simulink model "BFE_TestHarness"  (Simulink 8.6)
settings: Solver=FixedStepDiscrete  StartTime=0.0  StopTime=3  FixedStep=Ts  RelTol=1e-3
PreLoadFcn:
  | addpath('MBD_Tests')
  | 
  | load('Workspace\EnvVar.mat')
  | run('MBD_Tests\MBD_tests_init.m')
  | if exist('tl_preloadfcn','file'), tl_preloadfcn(gcs,402); end
PostLoadFcn:
  | if exist('tl_postloadfcn','file'), tl_postloadfcn(gcs,402); end
InitFcn:
  | if exist('tlds_init','file'), tlds_init(gcs); end
StartFcn:
  | if exist('tlds_start','file'), tlds_start(gcs); end
StopFcn:
  | if exist('tlds_stop','file'), tlds_stop(gcs); end
undefined symbols (not defined in the file): ddv, Ts, u2, u3, u4
libraries: tllib x11, simulink x8, LIB_TF_G_111 x2, LIB_TF_G_12_StepControl x2, LIB_TF_G_112 x1, LIB_TF_G_113 x1
(part 2 of 17)

== system BFE_TestHarness/BFE_AC_BeltFunctionExecution/Subsystem/BFE_AC_BeltFunctionExecution/BFE_AC_BeltFunctionExecution/BFE_runExecuteEmergencyBrakingSequence ==
  u8MotorStageStatus_in : Inport  PortDimensions=1  mask(TL_Inport){data={'autosar',{'useautosarcommunication',1,'kind',3,'interrunnablevariable','u8MotorStageStatus'},'date',736809.44014567125}}
      settings: CopyFcn=if exist('tl_reset_reviewflag','file')==2,tl_reset_reviewflag(gcbh);end  DeleteFcn=if exist('delete_tlblock','file')==2,delete_tlblock(gcbh);end  NameChangeFcn=if exist('rename_tlblock','file')==2,rename_tlblock(gcbh);end  OpenFcn=if exist('tl_open_blockdlg','file')==2,tl_open_blockdlg(gcbh);else,open_system(gcbh,'parameter');end
      mask Help: eval(['if exist(''tl_online_help'',''file'') == 2, tl_online_help(''Topic'',''TL_Inport''),else, web([''jar:file:///'',matlabroot,''/help/toolbox/simulink/help.jar!/slref/' lower(get_param(gcbh,'Blocktype')) '.html''], ''-helpbrowser''),end'])
      mask Display: plot([0.2 0.35 NaN 0.65 0.8],[0 1 NaN 0 1]);
  s16MotorPowerOrder : Inport  Port=2  PortDimensions=1  mask(TL_Inport){data={'autosar',{'useautosarcommunication',1,'kind',3,'interrunnablevariable','s16MotorPowerOrder'},'date',736809.44014613423}}
      settings: CopyFcn=if exist('tl_reset_reviewflag','file')==2,tl_reset_reviewflag(gcbh);end  DeleteFcn=if exist('delete_tlblock','file')==2,delete_tlblock(gcbh);end  NameChangeFcn=if exist('rename_tlblock','file')==2,rename_tlblock(gcbh);end  OpenFcn=if exist('tl_open_blockdlg','file')==2,tl_open_blockdlg(gcbh);else,open_system(gcbh,'parameter');end
      mask Help: eval(['if exist(''tl_online_help'',''file'') == 2, tl_online_help(''Topic'',''TL_Inport''),else, web([''jar:file:///'',matlabroot,''/help/toolbox/simulink/help.jar!/slref/' lower(get_param(gcbh,'Blocktype')) '.html''], ''-helpbrowser''),end'])
      mask Display: plot([0.2 0.35 NaN 0.65 0.8],[0 1 NaN 0 1]);
  SSCP_pclMotorCurrent_ReadMotorCurrentInmA : Inport  Port=3  PortDimensions=1  mask(TL_Inport){data={'autosar',{'useautosarcommunication',1,'kind',4,'clientserverport','pclMotor_I','operation','Get_mA'},'date',735951.66862153937}}
      settings: CopyFcn=if exist('tl_reset_reviewflag','file')==2,tl_reset_reviewflag(gcbh);end  DeleteFcn=if exist('delete_tlblock','file')==2,delete_tlblock(gcbh);end  NameChangeFcn=if exist('rename_tlblock','file')==2,rename_tlblock(gcbh);end  OpenFcn=if exist('tl_open_blockdlg','file')==2,tl_open_blockdlg(gcbh);else,open_system(gcbh,'parameter');end
      mask Help: eval(['if exist(''tl_online_help'',''file'') == 2, tl_online_help(''Topic'',''TL_Inport''),else, web([''jar:file:///'',matlabroot,''/help/toolbox/simulink/help.jar!/slref/' lower(get_param(gcbh,'Blocktype')) '.html''], ''-helpbrowser''),end'])
      mask Display: plot([0.2 0.35 NaN 0.65 0.8],[0 1 NaN 0 1]);
  Trigger : TriggerPort  RequirementInfo={} %GIDa_b93913d7_0985_4350_88c4_327c5b9b98e8  TriggerType=function-call
  ANG regulation : Subsystem  TreatAsAtomicUnit=on
  Constant : Constant  Value=ddv('Common/KU8_ONE')  mask(TL_Constant){data={'output',{'variable','Common/KU8_ONE'},'date',735951.66860753472}}
      settings: CopyFcn=if exist('tl_reset_reviewflag','file')==2,tl_reset_reviewflag(gcbh);end  DeleteFcn=if exist('delete_tlblock','file')==2,delete_tlblock(gcbh);end  NameChangeFcn=if exist('rename_tlblock','file')==2,rename_tlblock(gcbh);end  OpenFcn=if exist('tl_open_blockdlg','file')==2,tl_open_blockdlg(gcbh);else,open_system(gcbh,'parameter');end
      mask Help: eval(['if exist(''tl_online_help'',''file'') == 2, tl_online_help(''Topic'',''TL_Constant''),else, web([''jar:file:///'',matlabroot,''/help/toolbox/simulink/help.jar!/slref/' lower(get_param(gcbh,'Blocktype')) '.html''], ''-helpbrowser''),end'])
      mask Display: plot([-0.05, 1.05, NaN, -0.05, 1.05],[.01, .01, NaN, .99, .99])
  Constant1 : Constant  Value=ddv('EmergencyBraking/CAL_KU16_PYRO_SEQ_BRAKING_DURATION')  SampleTime=-1  mask(TL_Constant){data={'output',{'variable','EmergencyBraking/CAL_KU16_PYRO_SEQ_BRAKING_DURATION'},'date',735951.66860717593}}
      settings: CopyFcn=if exist('tl_reset_reviewflag','file')==2,tl_reset_reviewflag(gcbh);end  DeleteFcn=if exist('delete_tlblock','file')==2,delete_tlblock(gcbh);end  NameChangeFcn=if exist('rename_tlblock','file')==2,rename_tlblock(gcbh);end  OpenFcn=if exist('tl_open_blockdlg','file')==2,tl_open_blockdlg(gcbh);else,open_system(gcbh,'parameter');end
      mask Help: eval(['if exist(''tl_online_help'',''file'') == 2, tl_online_help(''Topic'',''TL_Constant''),else, web([''jar:file:///'',matlabroot,''/help/toolbox/simulink/help.jar!/slref/' lower(get_param(gcbh,'Blocktype')) '.html''], ''-helpbrowser''),end'])
      mask Display: plot([-0.05, 1.05, NaN, -0.05, 1.05],[.01, .01, NaN, .99, .99])
  Constant2 : Constant  Value=ddv('Common/KU16_ZERO')  mask(TL_Constant){data={'output',{'variable','Common/KU16_ZERO'},'date',735951.6686068055}}
      settings: CopyFcn=if exist('tl_reset_reviewflag','file')==2,tl_reset_reviewflag(gcbh);end  DeleteFcn=if exist('delete_tlblock','file')==2,delete_tlblock(gcbh);end  NameChangeFcn=if exist('rename_tlblock','file')==2,rename_tlblock(gcbh);end  OpenFcn=if exist('tl_open_blockdlg','file')==2,tl_open_blockdlg(gcbh);else,open_system(gcbh,'parameter');end
      mask Help: eval(['if exist(''tl_online_help'',''file'') == 2, tl_online_help(''Topic'',''TL_Constant''),else, web([''jar:file:///'',matlabroot,''/help/toolbox/simulink/help.jar!/slref/' lower(get_param(gcbh,'Blocktype')) '.html''], ''-helpbrowser''),end'])
      mask Display: plot([-0.05, 1.05, NaN, -0.05, 1.05],[.01, .01, NaN, .99, .99])
  Idle State : Subsystem  TreatAsAtomicUnit=on
  If : If  IfExpression=u1
  Relational Operator : RelationalOperator  Operator=~=  OutDataTypeStr=boolean  mask(TL_RelationalOperator){data={'date',735951.66860112268}}
      settings: DeleteFcn=if exist('delete_tlblock','file')==2,delete_tlblock(gcbh);end  NameChangeFcn=if exist('rename_tlblock','file')==2,rename_tlblock(gcbh);end  OpenFcn=if exist('tl_open_blockdlg','file')==2,tl_open_blockdlg(gcbh);else,open_system(gcbh,'parameter');end
      mask Help: eval(['if exist(''tl_online_help'',''file'') == 2, tl_online_help(''Topic'',''TL_RelationalOperator''),else, web([''jar:file:///'',matlabroot,''/help/toolbox/simulink/help.jar!/slref/' lower(get_param(gcbh,'Blocktype')) '.html''], ''-helpbrowser''),end'])
      mask Display: plot([-0.05, 1.05, NaN, -0.05, 1.05],[.01, .01, NaN, .99, .99])
  Relational Operator1 : RelationalOperator  Operator=>  OutDataTypeStr=boolean  mask(TL_RelationalOperator){data={'output',{'name','bIsFirstPhaseFinished'},'date',735951.66860086808}}
      settings: DeleteFcn=if exist('delete_tlblock','file')==2,delete_tlblock(gcbh);end  NameChangeFcn=if exist('rename_tlblock','file')==2,rename_tlblock(gcbh);end  OpenFcn=if exist('tl_open_blockdlg','file')==2,tl_open_blockdlg(gcbh);else,open_system(gcbh,'parameter');end
      mask Help: eval(['if exist(''tl_online_help'',''file'') == 2, tl_online_help(''Topic'',''TL_RelationalOperator''),else, web([''jar:file:///'',matlabroot,''/help/toolbox/simulink/help.jar!/slref/' lower(get_param(gcbh,'Blocktype')) '.html''], ''-helpbrowser''),end'])
      mask Display: plot([-0.05, 1.05, NaN, -0.05, 1.05],[.01, .01, NaN, .99, .99])
  Runnable : tllib/Function  data={'autosar',{'useautosarspecification',1,'softwarecomponent','AUTOLIV/SoftwareComponents/BFE/BFE_AC_BeltFunctionExecution','runnable','BFE_runExecuteEmergencyBrakingSequence'},'date',736809.44014254631}  displayString=RUNNABLE
  Sum : Sum  mask(TL_Sum){data={'output',{'name','u16LocalCounter','type','UInt16','checkmin',1,'checkmax',1},'date',735951.66860057868}}
      settings: CopyFcn=if exist('tl_reset_reviewflag','file')==2,tl_reset_reviewflag(gcbh);end  DeleteFcn=if exist('delete_tlblock','file')==2,delete_tlblock(gcbh);end  NameChangeFcn=if exist('rename_tlblock','file')==2,rename_tlblock(gcbh);end  OpenFcn=if exist('tl_open_blockdlg','file')==2,tl_open_blockdlg(gcbh);else,open_system(gcbh,'parameter');end
      mask Help: eval(['if exist(''tl_online_help'',''file'') == 2, tl_online_help(''Topic'',''TL_Sum''),else, web([''jar:file:///'',matlabroot,''/help/toolbox/simulink/help.jar!/slref/' lower(get_param(gcbh,'Blocktype')) '.html''], ''-helpbrowser''),end'])
      mask Display: plot([-0.05, 1.05, NaN, -0.05, 1.05],[.01, .01, NaN, .99, .99])
  Switch : Switch  Criteria=u2 ~= 0  mask(TL_Switch){data={'output',{'name','u16FilteredPrevCounterECPL','type','UInt16'},'date',735951.66860002314}}
      settings: CopyFcn=if exist('tl_reset_reviewflag','file')==2,tl_reset_reviewflag(gcbh);end  DeleteFcn=if exist('delete_tlblock','file')==2,delete_tlblock(gcbh);end  NameChangeFcn=if exist('rename_tlblock','file')==2,rename_tlblock(gcbh);end  OpenFcn=if exist('tl_open_blockdlg','file')==2,tl_open_blockdlg(gcbh);else,open_system(gcbh,'parameter');end
      mask Help: eval(['if exist(''tl_online_help'',''file'') == 2, tl_online_help(''Topic'',''TL_Switch''),else, web([''jar:file:///'',matlabroot,''/help/toolbox/simulink/help.jar!/slref/' lower(get_param(gcbh,'Blocktype')) '.html''], ''-helpbrowser''),end'])
      mask Display: plot([-0.05, 1.05, NaN, -0.05, 1.05],[.01, .01, NaN, .99, .99])
  Unit Delay : UnitDelay  SampleTime=-1  mask(TL_UnitDelay){data={'output',{'type','UInt16'},'state',{'name','u16CounterEmergencySeq','type','UInt16'},'date',735951.6685995023}}
      settings: CopyFcn=if exist('tl_reset_reviewflag','file')==2,tl_reset_reviewflag(gcbh);end  DeleteFcn=if exist('delete_tlblock','file')==2,delete_tlblock(gcbh);end  NameChangeFcn=if exist('rename_tlblock','file')==2,rename_tlblock(gcbh);end  OpenFcn=if exist('tl_open_blockdlg','file')==2,tl_open_blockdlg(gcbh);else,open_system(gcbh,'parameter');end
      mask Help: eval(['if exist(''tl_online_help'',''file'') == 2, tl_online_help(''Topic'',''TL_UnitDelay''),else, web([''jar:file:///'',matlabroot,''/help/toolbox/simulink/help.jar!/slref/' lower(get_param(gcbh,'Blocktype')) '.html''], ''-helpbrowser''),end'])
      mask Display: plot([-0.05, 1.05, NaN, -0.05, 1.05],[.01, .01, NaN, .99, .99])
  Unit Delay1 : UnitDelay  InitialCondition=170  SampleTime=-1  mask(TL_UnitDelay){data={'output',{'type','UInt8'},'state',{'name','u8PrevMotorStageStatus','type','UInt8'},'date',735951.66859895829}}
      settings: CopyFcn=if exist('tl_reset_reviewflag','file')==2,tl_reset_reviewflag(gcbh);end  DeleteFcn=if exist('delete_tlblock','file')==2,delete_tlblock(gcbh);end  NameChangeFcn=if exist('rename_tlblock','file')==2,rename_tlblock(gcbh);end  OpenFcn=if exist('tl_open_blockdlg','file')==2,tl_open_blockdlg(gcbh);else,open_system(gcbh,'parameter');end
      mask Help: eval(['if exist(''tl_online_help'',''file'') == 2, tl_online_help(''Topic'',''TL_UnitDelay''),else, web([''jar:file:///'',matlabroot,''/help/toolbox/simulink/help.jar!/slref/' lower(get_param(gcbh,'Blocktype')) '.html''], ''-helpbrowser''),end'])
      mask Display: plot([-0.05, 1.05, NaN, -0.05, 1.05],[.01, .01, NaN, .99, .99])
  terminator{2..5} (4 alike) : Terminator
  u8MotorStageStatus : Merge  mask(TL_Merge){data={'output',{'name','$B'},'date',735951.66859842592}}
      settings: CopyFcn=if exist('tl_reset_reviewflag','file')==2,tl_reset_reviewflag(gcbh);end  DeleteFcn=if exist('delete_tlblock','file')==2,delete_tlblock(gcbh);end  NameChangeFcn=if exist('rename_tlblock','file')==2,rename_tlblock(gcbh);end  OpenFcn=if exist('tl_open_blockdlg','file')==2,tl_open_blockdlg(gcbh);else,open_system(gcbh,'parameter');end
      mask Help: eval(['if exist(''tl_online_help'',''file'') == 2, tl_online_help(''Topic'',''TL_Merge''),else, web([''jar:file:///'',matlabroot,''/help/toolbox/simulink/help.jar!/slref/' lower(get_param(gcbh,'Blocktype')) '.html''], ''-helpbrowser''),end'])
      mask Display: plot([-0.05, 1.05, NaN, -0.05, 1.05],[.01, .01, NaN, .99, .99])
  u8MotorStageStatus_out : Outport  PortDimensions=1  InitialOutput=170  mask(TL_Outport){data={'autosar',{'useautosarcommunication',1,'kind',3,'communicationmode',1,'interrunnablevariable','u8MotorStageStatus'},'date',736809.4401464815}}
      settings: CopyFcn=if exist('tl_reset_reviewflag','file')==2,tl_reset_reviewflag(gcbh);end  DeleteFcn=if exist('delete_tlblock','file')==2,delete_tlblock(gcbh);end  NameChangeFcn=if exist('rename_tlblock','file')==2,rename_tlblock(gcbh);end  OpenFcn=if exist('tl_open_blockdlg','file')==2,tl_open_blockdlg(gcbh);else,open_system(gcbh,'parameter');end
      mask Help: eval(['if exist(''tl_online_help'',''file'') == 2, tl_online_help(''Topic'',''TL_Outport''),else, web([''jar:file:///'',matlabroot,''/help/toolbox/simulink/help.jar!/slref/' lower(get_param(gcbh,'Blocktype')) '.html''], ''-helpbrowser''),end'])
      mask Display: plot([0.2 0.35 NaN 0.65 0.8],[0 1 NaN 0 1]);
  wires:
  u8MotorStageStatus/1 -> u8MotorStageStatus_out/1
  Constant/1 -> Sum/1
  Constant1/1 -> Relational Operator1/1
  If/1 -> ANG regulation/Action
  Relational Operator1/1 -> If/1
  If/2 -> Idle State/Action
  Sum/1 -> Relational Operator1/2, Unit Delay/1
  Unit Delay/1 -> Switch/3
  s16MotorPowerOrder/1 -> Idle State/1(s16MotorPowerOrder), ANG regulation/2(s16MotorPowerOrder)
  SSCP_pclMotorCurrent_ReadMotorCurrentInmA/1 -> ANG regulation/1(u32MotorCurrent)
  Idle State/1(SSCP_pclMotorPowerOrder_SetPowerOrder) -> terminator2/1
  ANG regulation/1(SSCP_pclMotorPowerOrder_SetPowerOrder) -> terminator3/1
  Idle State/2(s16MotorPowerOrder1) -> terminator4/1
  ANG regulation/2(s16MotorPowerOrder1) -> terminator5/1
  Unit Delay1/1 -> Relational Operator/2
  Switch/1 -> Sum/2
  Relational Operator/1 -> Switch/2
  Constant2/1 -> Switch/1
  u8MotorStageStatus_in/1 -> Relational Operator/1, Unit Delay1/1
  ANG regulation/3(u8MotorStageStatus1) -> u8MotorStageStatus/1
  Idle State/3(u8MotorStageStatus1) -> u8MotorStageStatus/2

== system BFE_TestHarness/BFE_AC_BeltFunctionExecution/Subsystem/BFE_AC_BeltFunctionExecution/BFE_AC_BeltFunctionExecution/BFE_runExecuteHighPowerStep ==
  u16StepDuration : Inport  PortDimensions=1  mask(TL_Inport){data={'autosar',{'useautosarcommunication',1,'kind',3,'interrunnablevariable','u16StepDuration'},'date',736809.4401470602}}
      settings: CopyFcn=if exist('tl_reset_reviewflag','file')==2,tl_reset_reviewflag(gcbh);end  DeleteFcn=if exist('delete_tlblock','file')==2,delete_tlblock(gcbh);end  NameChangeFcn=if exist('rename_tlblock','file')==2,rename_tlblock(gcbh);end  OpenFcn=if exist('tl_open_blockdlg','file')==2,tl_open_blockdlg(gcbh);else,open_system(gcbh,'parameter');end
      mask Help: eval(['if exist(''tl_online_help'',''file'') == 2, tl_online_help(''Topic'',''TL_Inport''),else, web([''jar:file:///'',matlabroot,''/help/toolbox/simulink/help.jar!/slref/' lower(get_param(gcbh,'Blocktype')) '.html''], ''-helpbrowser''),end'])
      mask Display: plot([0.2 0.35 NaN 0.65 0.8],[0 1 NaN 0 1]);
  s32FirstOrderValue : Inport  Port=2  PortDimensions=1  mask(TL_Inport){data={'autosar',{'useautosarcommunication',1,'kind',3,'interrunnablevariable','s32FirstOrderValue'},'date',736809.44014717592}}
      settings: CopyFcn=if exist('tl_reset_reviewflag','file')==2,tl_reset_reviewflag(gcbh);end  DeleteFcn=if exist('delete_tlblock','file')==2,delete_tlblock(gcbh);end  NameChangeFcn=if exist('rename_tlblock','file')==2,rename_tlblock(gcbh);end  OpenFcn=if exist('tl_open_blockdlg','file')==2,tl_open_blockdlg(gcbh);else,open_system(gcbh,'parameter');end
      mask Help: eval(['if exist(''tl_online_help'',''file'') == 2, tl_online_help(''Topic'',''TL_Inport''),else, web([''jar:file:///'',matlabroot,''/help/toolbox/simulink/help.jar!/slref/' lower(get_param(gcbh,'Blocktype')) '.html''], ''-helpbrowser''),end'])
      mask Display: plot([0.2 0.35 NaN 0.65 0.8],[0 1 NaN 0 1]);
  u8OrderType : Inport  Port=3  PortDimensions=1  mask(TL_Inport){data={'autosar',{'useautosarcommunication',1,'kind',3,'interrunnablevariable','u8OrderType'},'date',736809.44014740735}}
      settings: CopyFcn=if exist('tl_reset_reviewflag','file')==2,tl_reset_reviewflag(gcbh);end  DeleteFcn=if exist('delete_tlblock','file')==2,delete_tlblock(gcbh);end  NameChangeFcn=if exist('rename_tlblock','file')==2,rename_tlblock(gcbh);end  OpenFcn=if exist('tl_open_blockdlg','file')==2,tl_open_blockdlg(gcbh);else,open_system(gcbh,'parameter');end
      mask Help: eval(['if exist(''tl_online_help'',''file'') == 2, tl_online_help(''Topic'',''TL_Inport''),else, web([''jar:file:///'',matlabroot,''/help/toolbox/simulink/help.jar!/slref/' lower(get_param(gcbh,'Blocktype')) '.html''], ''-helpbrowser''),end'])
      mask Display: plot([0.2 0.35 NaN 0.65 0.8],[0 1 NaN 0 1]);
  u8MotorStageStatus : Inport  Port=4  PortDimensions=1  mask(TL_Inport){data={'autosar',{'useautosarcommunication',1,'kind',3,'interrunnablevariable','u8MotorStageStatus'},'date',736809.44014752319}}
      settings: CopyFcn=if exist('tl_reset_reviewflag','file')==2,tl_reset_reviewflag(gcbh);end  DeleteFcn=if exist('delete_tlblock','file')==2,delete_tlblock(gcbh);end  NameChangeFcn=if exist('rename_tlblock','file')==2,rename_tlblock(gcbh);end  OpenFcn=if exist('tl_open_blockdlg','file')==2,tl_open_blockdlg(gcbh);else,open_system(gcbh,'parameter');end
      mask Help: eval(['if exist(''tl_online_help'',''file'') == 2, tl_online_help(''Topic'',''TL_Inport''),else, web([''jar:file:///'',matlabroot,''/help/toolbox/simulink/help.jar!/slref/' lower(get_param(gcbh,'Blocktype')) '.html''], ''-helpbrowser''),end'])
      mask Display: plot([0.2 0.35 NaN 0.65 0.8],[0 1 NaN 0 1]);
  s16MotorPowerOrder : Inport  Port=5  PortDimensions=1  mask(TL_Inport){data={'autosar',{'useautosarcommunication',1,'kind',3,'interrunnablevariable','s16MotorPowerOrder'},'date',736809.4401476389}}
      settings: CopyFcn=if exist('tl_reset_reviewflag','file')==2,tl_reset_reviewflag(gcbh);end  DeleteFcn=if exist('delete_tlblock','file')==2,delete_tlblock(gcbh);end  NameChangeFcn=if exist('rename_tlblock','file')==2,rename_tlblock(gcbh);end  OpenFcn=if exist('tl_open_blockdlg','file')==2,tl_open_blockdlg(gcbh);else,open_system(gcbh,'parameter');end
      mask Help: eval(['if exist(''tl_online_help'',''file'') == 2, tl_online_help(''Topic'',''TL_Inport''),else, web([''jar:file:///'',matlabroot,''/help/toolbox/simulink/help.jar!/slref/' lower(get_param(gcbh,'Blocktype')) '.html''], ''-helpbrowser''),end'])
      mask Display: plot([0.2 0.35 NaN 0.65 0.8],[0 1 NaN 0 1]);
  SSCP_pclVehicleAnalogSignals_GetBatteryVoltage : Inport  Port=6  PortDimensions=1  mask(TL_Inport){data={'autosar',{'useautosarcommunication',1,'kind',4,'clientserverport','pclKL30_V','operation','Get'},'date',735951.66859260411}}
      settings: CopyFcn=if exist('tl_reset_reviewflag','file')==2,tl_reset_reviewflag(gcbh);end  DeleteFcn=if exist('delete_tlblock','file')==2,delete_tlblock(gcbh);end  NameChangeFcn=if exist('rename_tlblock','file')==2,rename_tlblock(gcbh);end  OpenFcn=if exist('tl_open_blockdlg','file')==2,tl_open_blockdlg(gcbh);else,open_system(gcbh,'parameter');end
      mask Help: eval(['if exist(''tl_online_help'',''file'') == 2, tl_online_help(''Topic'',''TL_Inport''),else, web([''jar:file:///'',matlabroot,''/help/toolbox/simulink/help.jar!/slref/' lower(get_param(gcbh,'Blocktype')) '.html''], ''-helpbrowser''),end'])
      mask Display: plot([0.2 0.35 NaN 0.65 0.8],[0 1 NaN 0 1]);
  SSCP_pclMotorCurrent_ReadMotorCurrentInmA : Inport  Port=7  PortDimensions=1  mask(TL_Inport){data={'autosar',{'useautosarcommunication',1,'kind',4,'clientserverport','pclMotor_I','operation','Get_mA'},'date',735951.66859108792}}
      settings: CopyFcn=if exist('tl_reset_reviewflag','file')==2,tl_reset_reviewflag(gcbh);end  DeleteFcn=if exist('delete_tlblock','file')==2,delete_tlblock(gcbh);end  NameChangeFcn=if exist('rename_tlblock','file')==2,rename_tlblock(gcbh);end  OpenFcn=if exist('tl_open_blockdlg','file')==2,tl_open_blockdlg(gcbh);else,open_system(gcbh,'parameter');end
      mask Help: eval(['if exist(''tl_online_help'',''file'') == 2, tl_online_help(''Topic'',''TL_Inport''),else, web([''jar:file:///'',matlabroot,''/help/toolbox/simulink/help.jar!/slref/' lower(get_param(gcbh,'Blocktype')) '.html''], ''-helpbrowser''),end'])
      mask Display: plot([0.2 0.35 NaN 0.65 0.8],[0 1 NaN 0 1]);
  Trigger : TriggerPort  RequirementInfo={} %GIDa_67490f2f_d1af_406b_8dc1_b701e728c234  TriggerType=function-call
  HP Config Preprocessor : Constant  RequirementInfo={} %GIDa_4f0a43d1_5b42_442f_a84b_10ac092f983d  SampleTime=-1  mask(TL_Constant){data={'output',{'variable','BFE_Config_PreProc/BFE_CFG_OPT_HIGH_POWER'},'date',735951.66858878476}}
      settings: CopyFcn=if exist('tl_reset_reviewflag','file')==2,tl_reset_reviewflag(gcbh);end  DeleteFcn=if exist('delete_tlblock','file')==2,delete_tlblock(gcbh);end  NameChangeFcn=if exist('rename_tlblock','file')==2,rename_tlblock(gcbh);end  OpenFcn=if exist('tl_open_blockdlg','file')==2,tl_open_blockdlg(gcbh);else,open_system(gcbh,'parameter');end
      mask Help: eval(['if exist(''tl_online_help'',''file'') == 2, tl_online_help(''Topic'',''TL_Constant''),else, web([''jar:file:///'',matlabroot,''/help/toolbox/simulink/help.jar!/slref/' lower(get_param(gcbh,'Blocktype')) '.html''], ''-helpbrowser''),end'])
      mask Display: plot([-0.05, 1.05, NaN, -0.05, 1.05],[.01, .01, NaN, .99, .99])
  HP feature activated : Subsystem  TreatAsAtomicUnit=on
  Preprocessor IF : If  RequirementInfo={} %GIDa_f50f23b0_e1b5_47ae_a898_8a67fe69b69a  IfExpression=u1  ShowElse=off  mask(TL_PreProcessorIf){data={'mode',2,'date',735951.66841171298}}
      settings: DeleteFcn=if exist('delete_tlblock','file')==2,delete_tlblock(gcbh);end  NameChangeFcn=if exist('rename_tlblock','file')==2,rename_tlblock(gcbh);end  OpenFcn=if exist('tl_open_blockdlg','file')==2,tl_open_blockdlg(gcbh);else,open_system(gcbh,'parameter');end
      mask Help: eval(['if exist(''tl_online_help'',''file'') == 2, tl_online_help(''Topic'',''TL_PreProcessorIf''),else, web([''jar:file:///'',matlabroot,''/help/toolbox/simulink/help.jar!/slref/' lower(get_param(gcbh,'Blocktype')) '.html''], ''-helpbrowser''),end'])
      mask Display:
      | plot([-0.05, 1.05, NaN, -0.05, 1.05],[.01, .01, NaN, .99, .99])
      | 
      | port_label('input', 1, 'u1')
      | port_label('output',1,'#ifdef u1');
  Runnable : tllib/Function  data={'autosar',{'useautosarspecification',1,'softwarecomponent','AUTOLIV/SoftwareComponents/BFE/BFE_AC_BeltFunctionExecution','runnable','BFE_runExecuteHighPowerStep'},'date',736809.44014277775}  displayString=RUNNABLE
  terminator2 : Terminator
  wires:
  u8MotorStageStatus/1 -> terminator2/1
  HP Config Preprocessor/1 -> Preprocessor IF/1
  Preprocessor IF/1 -> HP feature activated/Action
  u16StepDuration/1 -> HP feature activated/6(u16StepDuration)
  s32FirstOrderValue/1 -> HP feature activated/5(s32FirstOrderValue)
  SSCP_pclVehicleAnalogSignals_GetBatteryVoltage/1 -> HP feature activated/1(u16BatteryVoltage)
  SSCP_pclMotorCurrent_ReadMotorCurrentInmA/1 -> HP feature activated/4(u32MotorCurrentInmA)
  s16MotorPowerOrder/1 -> HP feature activated/3(s16MotorPowerOrder)
  u8OrderType/1 -> HP feature activated/2(u8OrderType)

== system BFE_TestHarness/BFE_AC_BeltFunctionExecution/Subsystem/BFE_AC_BeltFunctionExecution/BFE_AC_BeltFunctionExecution/BFE_runExecuteStandardSteps ==
  s32FirstOrderValue : Inport  PortDimensions=1  mask(TL_Inport){data={'autosar',{'useautosarcommunication',1,'kind',3,'interrunnablevariable','s32FirstOrderValue'},'date',736809.44014810189}}
      settings: CopyFcn=if exist('tl_reset_reviewflag','file')==2,tl_reset_reviewflag(gcbh);end  DeleteFcn=if exist('delete_tlblock','file')==2,delete_tlblock(gcbh);end  NameChangeFcn=if exist('rename_tlblock','file')==2,rename_tlblock(gcbh);end  OpenFcn=if exist('tl_open_blockdlg','file')==2,tl_open_blockdlg(gcbh);else,open_system(gcbh,'parameter');end
      mask Help: eval(['if exist(''tl_online_help'',''file'') == 2, tl_online_help(''Topic'',''TL_Inport''),else, web([''jar:file:///'',matlabroot,''/help/toolbox/simulink/help.jar!/slref/' lower(get_param(gcbh,'Blocktype')) '.html''], ''-helpbrowser''),end'])
      mask Display: plot([0.2 0.35 NaN 0.65 0.8],[0 1 NaN 0 1]);
  u8OrderType : Inport  Port=2  PortDimensions=1  mask(TL_Inport){data={'autosar',{'useautosarcommunication',1,'kind',3,'interrunnablevariable','u8OrderType'},'date',736809.4401482176}}
      settings: CopyFcn=if exist('tl_reset_reviewflag','file')==2,tl_reset_reviewflag(gcbh);end  DeleteFcn=if exist('delete_tlblock','file')==2,delete_tlblock(gcbh);end  NameChangeFcn=if exist('rename_tlblock','file')==2,rename_tlblock(gcbh);end  OpenFcn=if exist('tl_open_blockdlg','file')==2,tl_open_blockdlg(gcbh);else,open_system(gcbh,'parameter');end
      mask Help: eval(['if exist(''tl_online_help'',''file'') == 2, tl_online_help(''Topic'',''TL_Inport''),else, web([''jar:file:///'',matlabroot,''/help/toolbox/simulink/help.jar!/slref/' lower(get_param(gcbh,'Blocktype')) '.html''], ''-helpbrowser''),end'])
      mask Display: plot([0.2 0.35 NaN 0.65 0.8],[0 1 NaN 0 1]);
  s32OrderIncrementValue : Inport  Port=3  PortDimensions=1  mask(TL_Inport){data={'autosar',{'useautosarcommunication',1,'kind',3,'interrunnablevariable','s32OrderIncrementValue'},'date',736809.44014833332}}
      settings: CopyFcn=if exist('tl_reset_reviewflag','file')==2,tl_reset_reviewflag(gcbh);end  DeleteFcn=if exist('delete_tlblock','file')==2,delete_tlblock(gcbh);end  NameChangeFcn=if exist('rename_tlblock','file')==2,rename_tlblock(gcbh);end  OpenFcn=if exist('tl_open_blockdlg','file')==2,tl_open_blockdlg(gcbh);else,open_system(gcbh,'parameter');end
      mask Help: eval(['if exist(''tl_online_help'',''file'') == 2, tl_online_help(''Topic'',''TL_Inport''),else, web([''jar:file:///'',matlabroot,''/help/toolbox/simulink/help.jar!/slref/' lower(get_param(gcbh,'Blocktype')) '.html''], ''-helpbrowser''),end'])
      mask Display: plot([0.2 0.35 NaN 0.65 0.8],[0 1 NaN 0 1]);
  u8MotorStageStatus : Inport  Port=4
  s16MotorPowerOrder : Inport  Port=5  PortDimensions=1  mask(TL_Inport){data={'autosar',{'useautosarcommunication',1,'kind',3,'interrunnablevariable','s16MotorPowerOrder'},'date',736809.44014844904}}
      settings: CopyFcn=if exist('tl_reset_reviewflag','file')==2,tl_reset_reviewflag(gcbh);end  DeleteFcn=if exist('delete_tlblock','file')==2,delete_tlblock(gcbh);end  NameChangeFcn=if exist('rename_tlblock','file')==2,rename_tlblock(gcbh);end  OpenFcn=if exist('tl_open_blockdlg','file')==2,tl_open_blockdlg(gcbh);else,open_system(gcbh,'parameter');end
      mask Help: eval(['if exist(''tl_online_help'',''file'') == 2, tl_online_help(''Topic'',''TL_Inport''),else, web([''jar:file:///'',matlabroot,''/help/toolbox/simulink/help.jar!/slref/' lower(get_param(gcbh,'Blocktype')) '.html''], ''-helpbrowser''),end'])
      mask Display: plot([0.2 0.35 NaN 0.65 0.8],[0 1 NaN 0 1]);
  SSCP_pclMotorCurrent_ReadMotorCurrentInmA : Inport  Port=6  PortDimensions=1  mask(TL_Inport){data={'autosar',{'useautosarcommunication',1,'kind',4,'clientserverport','pclMotor_I','operation','Get_mA'},'date',735951.66840858792}}
      settings: CopyFcn=if exist('tl_reset_reviewflag','file')==2,tl_reset_reviewflag(gcbh);end  DeleteFcn=if exist('delete_tlblock','file')==2,delete_tlblock(gcbh);end  NameChangeFcn=if exist('rename_tlblock','file')==2,rename_tlblock(gcbh);end  OpenFcn=if exist('tl_open_blockdlg','file')==2,tl_open_blockdlg(gcbh);else,open_system(gcbh,'parameter');end
      mask Help: eval(['if exist(''tl_online_help'',''file'') == 2, tl_online_help(''Topic'',''TL_Inport''),else, web([''jar:file:///'',matlabroot,''/help/toolbox/simulink/help.jar!/slref/' lower(get_param(gcbh,'Blocktype')) '.html''], ''-helpbrowser''),end'])
      mask Display: plot([0.2 0.35 NaN 0.65 0.8],[0 1 NaN 0 1]);
  SSCP_pclVehicleAnalogSignals_GetBatteryVoltage : Inport  Port=7  PortDimensions=1  mask(TL_Inport){data={'autosar',{'useautosarcommunication',1,'kind',4,'clientserverport','pclKL30_V','operation','Get_2ms'},'date',735977.59735841432}}
      settings: CopyFcn=if exist('tl_reset_reviewflag','file')==2,tl_reset_reviewflag(gcbh);end  DeleteFcn=if exist('delete_tlblock','file')==2,delete_tlblock(gcbh);end  NameChangeFcn=if exist('rename_tlblock','file')==2,rename_tlblock(gcbh);end  OpenFcn=if exist('tl_open_blockdlg','file')==2,tl_open_blockdlg(gcbh);else,open_system(gcbh,'parameter');end
      mask Help: eval(['if exist(''tl_online_help'',''file'') == 2, tl_online_help(''Topic'',''TL_Inport''),else, web([''jar:file:///'',matlabroot,''/help/toolbox/simulink/help.jar!/slref/' lower(get_param(gcbh,'Blocktype')) '.html''], ''-helpbrowser''),end'])
      mask Display: plot([0.2 0.35 NaN 0.65 0.8],[0 1 NaN 0 1]);
  Trigger : TriggerPort  RequirementInfo={} %GIDa_8a9d6a75_7b35_403d_86e2_680b96bf35ca  TriggerType=function-call
  Bitwise Operator1 : tllib/Bitwise Operator  RequirementInfo={} %GIDa_b3a06111_65b0_4dd7_9ee5_ce11c796bc53  logicop=AND  UseBitMask=off  NumInputPorts=2  BitMask=bin2dec('11011001')  BitMaskRealWorld=Stored Integer  data={'date',735951.66840643517}
  ExecuteStandardSteps : Subsystem  RequirementInfo={} %GIDa_8da1e9c1_4c64_4b63_96ae_9e41ef9f12e5  TreatAsAtomicUnit=on
  If : If  RequirementInfo={} %GIDa_f9656b55_4671_45d1_a0d7_b30dde6b4010  IfExpression=u1==0  ShowElse=off
  KU8_ORDER_HIGH_POWER : Constant  RequirementInfo={} %GIDa_27445266_a7f6_49aa_b7be_da0e5d31f62d  Value=ddv('RTE_Define/KU8_ORDER_HIGH_POWER')  OutDataTypeStr=uint8  mask(TL_Constant){data={'output',{'variable','RTE_Define/KU8_ORDER_HIGH_POWER'},'date',735951.66850177082}}
      settings: CopyFcn=if exist('tl_reset_reviewflag','file')==2,tl_reset_reviewflag(gcbh);end  DeleteFcn=if exist('delete_tlblock','file')==2,delete_tlblock(gcbh);end  NameChangeFcn=if exist('rename_tlblock','file')==2,rename_tlblock(gcbh);end  OpenFcn=if exist('tl_open_blockdlg','file')==2,tl_open_blockdlg(gcbh);else,open_system(gcbh,'parameter');end
      mask Help: eval(['if exist(''tl_online_help'',''file'') == 2, tl_online_help(''Topic'',''TL_Constant''),else, web([''jar:file:///'',matlabroot,''/help/toolbox/simulink/help.jar!/slref/' lower(get_param(gcbh,'Blocktype')) '.html''], ''-helpbrowser''),end'])
      mask Display: plot([-0.05, 1.05, NaN, -0.05, 1.05],[.01, .01, NaN, .99, .99])
  Rescaler : DataTypeConversion  RequirementInfo={} %GIDa_30d1871e_9244_4b41_a49c_11d8ea8684c3  SaturateOnIntegerOverflow=on  RndMeth=Zero  mask(TL_Rescaler){data={'output',{'type','UInt8'},'date',735951.66850141203}}
      settings: DeleteFcn=if exist('delete_tlblock','file')==2,delete_tlblock(gcbh);end  NameChangeFcn=if exist('rename_tlblock','file')==2,rename_tlblock(gcbh);end  OpenFcn=if exist('tl_open_blockdlg','file')==2,tl_open_blockdlg(gcbh);else,open_system(gcbh,'parameter');end
      mask Help: eval(['if exist(''tl_online_help'',''file'') == 2, tl_online_help(''Topic'',''TL_Rescaler''),else, web([''jar:file:///'',matlabroot,''/help/toolbox/simulink/help.jar!/slref/' lower(get_param(gcbh,'Blocktype')) '.html''], ''-helpbrowser''),end'])
      mask Display: plot([-0.05, 1.05, NaN, -0.05, 1.05],[.01, .01, NaN, .99, .99])
  Rescaler1 : DataTypeConversion  SaturateOnIntegerOverflow=on  RndMeth=Zero  mask(TL_Rescaler){data={'output',{'name','s16PrevMotorCommand2ms'},'date',735951.66850109957}}
      settings: DeleteFcn=if exist('delete_tlblock','file')==2,delete_tlblock(gcbh);end  NameChangeFcn=if exist('rename_tlblock','file')==2,rename_tlblock(gcbh);end  OpenFcn=if exist('tl_open_blockdlg','file')==2,tl_open_blockdlg(gcbh);else,open_system(gcbh,'parameter');end
      mask Help: eval(['if exist(''tl_online_help'',''file'') == 2, tl_online_help(''Topic'',''TL_Rescaler''),else, web([''jar:file:///'',matlabroot,''/help/toolbox/simulink/help.jar!/slref/' lower(get_param(gcbh,'Blocktype')) '.html''], ''-helpbrowser''),end'])
      mask Display: plot([-0.05, 1.05, NaN, -0.05, 1.05],[.01, .01, NaN, .99, .99])
  Runnable : tllib/Function  data={'autosar',{'useautosarspecification',1,'softwarecomponent','AUTOLIV/SoftwareComponents/BFE/BFE_AC_BeltFunctionExecution','runnable','BFE_runExecuteStandardSteps'},'date',736809.4401430093}  displayString=RUNNABLE
  Unit Delay : UnitDelay  RequirementInfo={} %GIDa_c0584e06_e774_4214_9304_5300ebbd263f  SampleTime=-1  mask(TL_UnitDelay){data={'output',{'type','Bool'},'state',{'type','Bool'},'date',735951.6685007523}}
      settings: CopyFcn=if exist('tl_reset_reviewflag','file')==2,tl_reset_reviewflag(gcbh);end  DeleteFcn=if exist('delete_tlblock','file')==2,delete_tlblock(gcbh);end  NameChangeFcn=if exist('rename_tlblock','file')==2,rename_tlblock(gcbh);end  OpenFcn=if exist('tl_open_blockdlg','file')==2,tl_open_blockdlg(gcbh);else,open_system(gcbh,'parameter');end
      mask Help: eval(['if exist(''tl_online_help'',''file'') == 2, tl_online_help(''Topic'',''TL_UnitDelay''),else, web([''jar:file:///'',matlabroot,''/help/toolbox/simulink/help.jar!/slref/' lower(get_param(gcbh,'Blocktype')) '.html''], ''-helpbrowser''),end'])
      mask Display: plot([-0.05, 1.05, NaN, -0.05, 1.05],[.01, .01, NaN, .99, .99])
  wires:
  If/1 -> ExecuteStandardSteps/Action
  Bitwise Operator1/1 -> If/1, Unit Delay/1
  KU8_ORDER_HIGH_POWER/1 -> Bitwise Operator1/1
  Rescaler/1 -> Bitwise Operator1/2
  u8OrderType/1 -> Rescaler/1, ExecuteStandardSteps/3(u8OrderType)
  Unit Delay/1 -> ExecuteStandardSteps/7(bIsPrevStepHP)
  s16MotorPowerOrder/1 -> Rescaler1/1
  SSCP_pclVehicleAnalogSignals_GetBatteryVoltage/1 -> ExecuteStandardSteps/1(OA_pclVehicleAnalogSignals_GetBatteryVoltage)
  SSCP_pclMotorCurrent_ReadMotorCurrentInmA/1 -> ExecuteStandardSteps/2(OA_pclMotorCurrent_ReadMotorCurrentInmA)
  s32FirstOrderValue/1 -> ExecuteStandardSteps/4(s32FirstOrderValue)
  s32OrderIncrementValue/1 -> ExecuteStandardSteps/5(s32OrderIncrementValue)
  u8MotorStageStatus/1 -> ExecuteStandardSteps/8(u8MotorStageStatus)
  Rescaler1/1 -> ExecuteStandardSteps/6(s16OldPwm)

== system BFE_TestHarness/BFE_AC_BeltFunctionExecution/Subsystem/BFE_AC_BeltFunctionExecution/BFE_AC_BeltFunctionExecution/BFE_runResetMotorStageStatus ==
  Trigger : TriggerPort  RequirementInfo={} %GIDa_9727c40c_922b_4e17_8605_e58b349643bf  TriggerType=function-call
  Runnable : tllib/Function  data={'autosar',{'useautosarspecification',1,'softwarecomponent','AUTOLIV/SoftwareComponents/BFE/BFE_AC_BeltFunctionExecution','runnable','BFE_runResetMotorStageStatus'},'date',736809.44014324073}  displayString=RUNNABLE
  Src : Subsystem
  u8MotorStageStatus1 : Outport  PortDimensions=1  InitialOutput=170  mask(TL_Outport){data={'autosar',{'useautosarcommunication',1,'kind',3,'interrunnablevariable','u8MotorStageStatus'},'date',736809.44014902774}}
      settings: CopyFcn=if exist('tl_reset_reviewflag','file')==2,tl_reset_reviewflag(gcbh);end  DeleteFcn=if exist('delete_tlblock','file')==2,delete_tlblock(gcbh);end  NameChangeFcn=if exist('rename_tlblock','file')==2,rename_tlblock(gcbh);end  OpenFcn=if exist('tl_open_blockdlg','file')==2,tl_open_blockdlg(gcbh);else,open_system(gcbh,'parameter');end
      mask Help: eval(['if exist(''tl_online_help'',''file'') == 2, tl_online_help(''Topic'',''TL_Outport''),else, web([''jar:file:///'',matlabroot,''/help/toolbox/simulink/help.jar!/slref/' lower(get_param(gcbh,'Blocktype')) '.html''], ''-helpbrowser''),end'])
      mask Display: plot([0.2 0.35 NaN 0.65 0.8],[0 1 NaN 0 1]);
  wires:
  Src/1(u8MotorStageStatus) -> u8MotorStageStatus1/1
